simulink model "step5_setup_obsservor_test1"  (R2021b)
settings: Solver=FixedStepAuto  StartTime=0.0  StopTime=RunTime  FixedStep=time_step  RelTol=1e-3  EnableMultiTasking=on
values from neighbouring files (symbols this model uses):
  A = [0 1 0 0 ... (first row only)    [linearize_script.m]    (also in step4_0_linearize_operating_point.m = double(A); step4_linearized_system.mat = [0 0.306815158551 0 -109.913929424 0 1 -60.0152130057 0 126.; syms_test.m = double(A))
  adingain = [adin_gain 1 1 1 1 1]    [hwinit.m]    (also in hwinit_raw.m)
  adinoffs = [-adin_offs 0 0 0 0 0]    [hwinit.m]    (also in hwinit_raw.m = [adin_offs 0 0 0 0 0])
  B = [0 ... (first row only)    [linearize_script.m]    (also in step4_0_linearize_operating_point.m = double(B); step4_linearized_system.mat = [0 0 0 0 858.38566108]; syms_test.m = double(B))
  C = [1 0 0 0 ... (first row only)    [linearize_script.m]    (also in matrixmaker_linearization.m = [b_1_0 - P_3 * theta_d_2 * sin(theta_2)  -P_3 * (theta_d_1 +; step4_0_linearize_operating_point.m = [1 0 0 0 0; step4_linearized_system.mat = [1  0  0  0  0; 0  0  1  0  0]; syms_test.m)
  D = zeros(2,1)    [linearize_script.m]    (also in step4_0_linearize_operating_point.m; step4_linearized_system.mat = [0 0]; syms_test.m)
  daoutgain = 1*[-6]    [hwinit.m]    (also in hwinit_raw.m)
  daoutoffs = [0.00]    [hwinit.m]    (also in hwinit_raw.m)
  h = 0.001    [hwinit.m]    (also in hwinit_raw.m; init_fugi.m = fugiboard('Open', 'Pendulum1'); one_run.m = fugiboard('Open', 'pendulum1'); one_single_run.m = fugiboard('Open', 'pendulum1'))
  Ke = [179.790705396  -8.75441408307; 5045.03078547  -772.04516784; 51.075965998  222.058501149; 11187.8023059  11882.0258122; 15540.4857139  -3050.79062386]    [step5_observor.mat]    (also in step5_observor_design.m = place(A_, B_, 0.5*J)')
settings Model: Creator=rbabuska  LastModifiedBy=lyitingli
settings SolverCC: AlgebraicLoopSolver=TrustRegion
settings DataIOCC: LimitDataPoints=on  SaveFormat=Array  ReturnWorkspaceOutputs=off  SignalLoggingName=sigsOut
settings OptimizationCC: BooleanDataType=off  ExpressionDepthLimit=2147483647  InitFltsAndDblsToZero=on  LifeSpan=inf
settings DebuggingCC: SaveWithParameterizedLinksMsg=none  SignalResolutionControl=TryResolveAllWithWarning  MultiTaskDSMMsg=warning  MultiTaskCondExecSysMsg=none  AllowSymbolicDim=off  StateNameClashWarn=warning  SFUnexpectedBacktrackingDiag=warning  SFNoUnconditionalDefaultTransitionDiag=warning  SFExecutionAtInitializationDiag=none  SFMachineParentedDataDiag=warning  ArithmeticOperatorsInVariantConditions=warning
settings HardwareCC: ProdBitPerPointer=32  ProdBitPerSizeT=32  ProdBitPerPtrDiffT=32  ProdLargestAtomicFloat=None  ProdIntDivRoundTo=Undefined  ProdEndianess=Unspecified  ProdWordSize=32  ProdHWDeviceType=32-bit Generic  TargetUnknown=on
settings ModelReferenceCC: PropagateSignalLabelsOutOfModel=off
settings SFSimCC: SimUseLocalCustomCode=off  CustomCodeUndefinedFunction=UseInterfaceOnly
settings RTWCC: RTWUseLocalCustomCode=off
settings CodeAppCC: StateflowObjectComments=on
settings GRTTargetCC: TargetFcnLib=ansi_tfl_tmw.mat  TargetLangStandard=C89/C90 (ANSI)  CombineOutputUpdateFcns=off  GRTInterface=on
settings ConfigComp: CovMetricSettings=dw  CovSaveCumulativeToWorkspaceVar=on  CovSaveSingleToWorkspaceVar=on  CovExternalEMLEnable=off

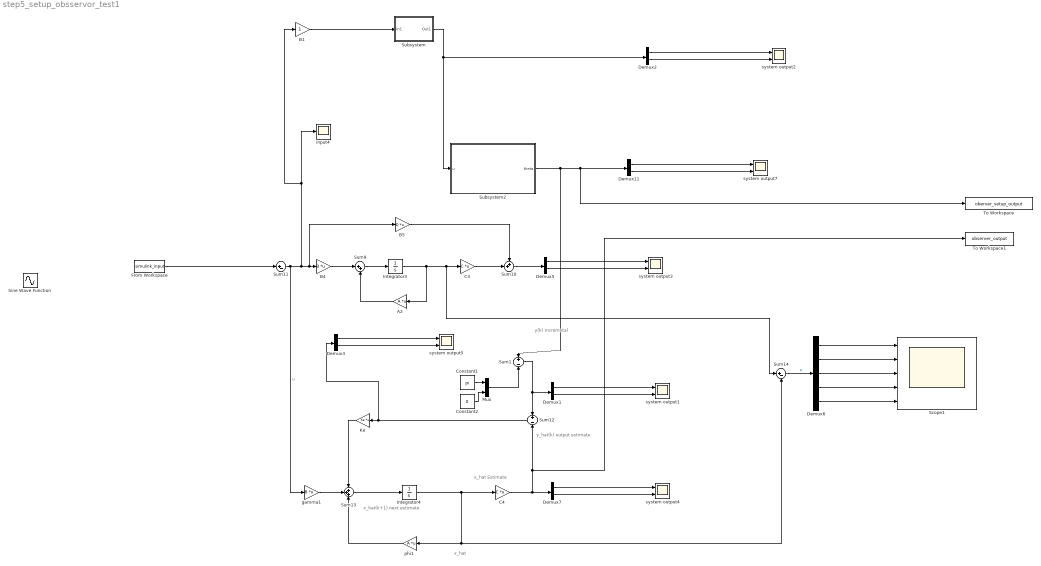
== system step5_setup_obsservor_test1 ==
  note: y_hat(k)
      | output estimate
  note: x_hat(k+1)
      | next estimate
  note: y(k)
      | incremetal
  note: x_hat
      | Estimate
  note: x_hat
  A2 : Gain  Gain=A  Multiplication=Matrix(K*u) (u vector)
  B1 : Gain
  B4 : Gain  Gain=B  Multiplication=Matrix(K*u)
  B5 : Gain  Gain=D  Multiplication=Matrix(K*u)
  C3 : Gain  Gain=C  Multiplication=Matrix(K*u) (u vector)
  C4 : Gain  Gain=C  Multiplication=Matrix(K*u) (u vector)
  Constant1 : Constant  Value=pi  SampleTime=-1
  Constant2 : Constant  Value=0  SampleTime=-1
  Demux{1..3,5,7,11} (6 alike) : Demux  Outputs=2
  Demux6 : Demux  Outputs=5
  From Workspace : FromWorkspace  SampleTime=-1
  Integrator3 : Integrator  InitialCondition=[0; 0; 0; 0; 0]
  Integrator4 : Integrator  InitialCondition=[0; 0; 0; 0; 0]
  Ke : Gain  Gain=Ke  Multiplication=Matrix(K*u) (u vector)
  Mux : Mux  Inputs=2
  Scope1 : Scope  NumInputPorts=5
  Sine Wave Function : Sin  Amplitude=1.5  Frequency=2*pi*2  SampleTime=0.001
  Subsystem : Subsystem
      mask Display: disp('Rotational\nPendulum')
  Subsystem2 : Subsystem
  Sum1 : Sum  Inputs=+|-
  Sum10 : Sum  Inputs=++|
  Sum11 : Sum  Inputs=|+-
  Sum12 : Sum  Inputs=+|-
  Sum13 : Sum  Inputs=+++
  Sum14 : Sum  Inputs=|+-
  Sum9 : Sum  Inputs=|++
  To Workspace : ToWorkspace  VariableName=oberver_setup_output  SampleTime=0.001
  To Workspace1 : ToWorkspace  VariableName=observer_output  SampleTime=0.001
  gamma1 : Gain  Gain=B  Multiplication=Matrix(K*u)
  input4 : Scope
  phi1 : Gain  Gain=A  Multiplication=Matrix(K*u) (u vector)
  system output{1..5,7} (6 alike) : Scope  NumInputPorts=2
  wires:
  Sum14/1 -> Demux6/1  "u"
  From Workspace/1 -> Sum11/1
  Sum10/1 -> Demux5/1
  Integrator3/1 -> C3/1, Sum14/1, A2/1
  Sum9/1 -> Integrator3/1
  Demux7/1 -> system output4/1
  Demux5/2 -> system output3/2
  Ke/1 -> Sum13/1
  B4/1 -> Sum9/1
  phi1/1 -> Sum13/3
  Demux5/1 -> system output3/1
  Demux6/3 -> Scope1/3
  Demux7/2 -> system output4/2
  Demux6/5 -> Scope1/5
  B5/1 -> Sum10/1
  A2/1 -> Sum9/2
  Demux6/4 -> Scope1/4
  Sum13/1 -> Integrator4/1
  Demux11/2 -> system output7/2
  Demux6/1 -> Scope1/1
  Integrator4/1 -> phi1/1, Sum14/2, C4/1
  gamma1/1 -> Sum13/2
  Sum11/1 -> B1/1, input4/1, B4/1, B5/1, gamma1/1  "u"
  C3/1 -> Sum10/2
  Demux11/1 -> system output7/1
  Demux6/2 -> Scope1/2
  Sum1/1 -> Demux1/1, Sum12/1
  Constant1/1 -> Mux/1
  Constant2/1 -> Mux/2
  Demux1/1 -> system output1/1
  Demux1/2 -> system output1/2
  Mux/1 -> Sum1/2
  Demux2/2 -> system output2/2
  Demux2/1 -> system output2/1
  Subsystem/1(Out1) -> Demux2/1, Subsystem2/1(u)
  B1/1 -> Subsystem/1(In1)
  Demux3/1 -> system output5/1
  Demux3/2 -> system output5/2
  Sum12/1 -> Demux3/1, Ke/1
  C4/1 -> To Workspace1/1, Sum12/2, Demux7/1
  Subsystem2/1(theta) -> Sum1/1, To Workspace/1, Demux11/1

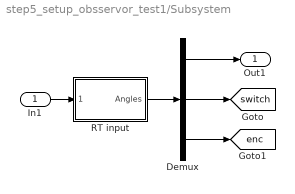
== system step5_setup_obsservor_test1/Subsystem ==
  In1 : Inport
  Demux : Demux  Outputs=[2 4 1]
  RT input : Subsystem  mask{Ts=h, channels=[6 7]}
      mask prompts: Ts "Sample time [s]:"; channels "Channels to read (e.g., [6 7])"
      mask init:
      | hwinit;
      | 
      | % initialize FPGA
      | fugihandle = fugiboard('Open', 'Pendulum1');
      | fugihandle.WatchdogTimeout = 0.5;
      | fugiboard('SetParams', fugihandle);
      | fugiboard('Write', fugihandle, 0, 0, 0, 0);  % dummy write to sync interface board
      | fugiboard('Write', fugihandle, 5, 1, 0, 0);  % reset position, activate relay
      | data = fugiboard('Read', fugihandle);        % get version info from FPGA
      | % model = bitshift(data(1), -5); 
      | % version = bitand(data(1), 31);
      | % disp(sprintf('FPGA setup %d, version %d', model, version)); % for the B&P it should say 1 1, or else there is a problem
      | fugiboard('Write', fugihandle, 0, 1, 0, 0);  % end reset
      | pause(0.1);                         % give relay some time to respond
      mask Display: disp('Rotational\nPendulum')
  Out1 : Outport
  tag scope: enc=global, switch=global
  wires:
  RT input/1(Angles) -> Demux/1
  Demux/1 -> Out1/1
  Demux/2 -> [switch]
  Demux/3 -> [enc]
  In1/1 -> RT input/1(Motors)

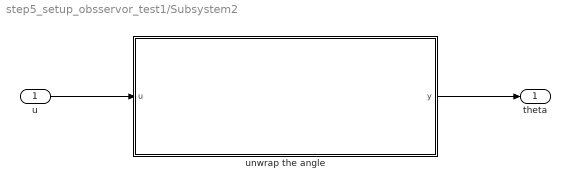
== system step5_setup_obsservor_test1/Subsystem2 ==
  u : Inport
  unwrap the angle : MATLAB Function  TreatAsAtomicUnit=on
  theta : Outport
  wires:
  u/1 -> unwrap the angle/1(u)
  unwrap the angle/1(y) -> theta/1

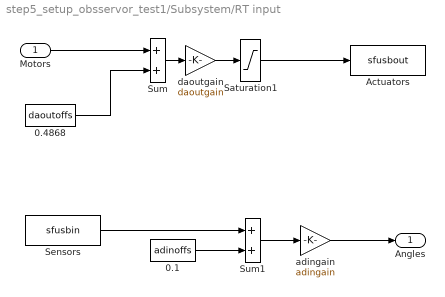
== system step5_setup_obsservor_test1/Subsystem/RT input ==
  Motors : Inport
  0.1 : Constant  Value=adinoffs
  0.4868 : Constant  Value=daoutoffs
  Actuators : S-Function  FunctionName=sfusbout  Parameters=Ts, fugihandle  SFunctionDeploymentMode=off  EnableBusSupport=off
  Saturation1 : Saturate  UpperLimit=10  LowerLimit=-10
  Sensors : S-Function  FunctionName=sfusbin  Parameters=Ts, fugihandle, channels  SFunctionDeploymentMode=off  EnableBusSupport=off
  Sum : Sum  InputSameDT=on  SaturateOnIntegerOverflow=on  OutDataTypeStr=Inherit: Same as first input
  Sum1 : Sum  InputSameDT=on  SaturateOnIntegerOverflow=on  OutDataTypeStr=Inherit: Same as first input
  adingain : Gain  Gain=adingain  SaturateOnIntegerOverflow=on  OutDataTypeStr=Inherit: Same as input  ParamDataTypeStr=Inherit: Same as input
  daoutgain : Gain  Gain=daoutgain  SaturateOnIntegerOverflow=on  OutDataTypeStr=Inherit: Same as input  ParamDataTypeStr=Inherit: Same as input
  Angles : Outport
  wires:
  Sum/1 -> daoutgain/1
  0.4868/1 -> Sum/2
  Motors/1 -> Sum/1
  Sum1/1 -> adingain/1
  0.1/1 -> Sum1/2
  adingain/1 -> Angles/1
  Saturation1/1 -> Actuators/1
  daoutgain/1 -> Saturation1/1
  Sensors/1 -> Sum1/1

== matlab function step5_setup_obsservor_test1/Subsystem2/unwrap the angle ==
  settings: updateMethod=DISCRETE  sampleTime=0.001
  data: u input size=2; y output size=2
function y = unwrap_angle(u)

y = unwrap(u);
% y = u;
